simulink model "problem1_model"  (R2023b)
settings: Solver=ode8  StartTime=0.0  StopTime=30  FixedStep=1e-3  RelTol=1e-3
values from neighbouring files (symbols this model uses):
  h = A_3    (= 2)    [plotting_from_sim.m]    (also in problem1.m; problem1_1.m; proj_cnl_exer_21.m = x1-x2)
  ic = 0    [plotting_from_sim.m]    (also in problem1.m; problem1_1.m)
  k = 2    [plotting_from_sim.m]    (also in problem1.m; problem1_1.m)
  M_2 = 1    [plotting_from_sim.m]    (also in problem1.m; problem1_1.m)
  M_3 = B_3    (= 0.5)    [plotting_from_sim.m]    (also in problem1.m; problem1_1.m)
  S_1 = A_1    (= 0.5)    [plotting_from_sim.m]    (also in problem1.m; problem1_1.m)
  S_2 = A_2    (= 1)    [plotting_from_sim.m]    (also in problem1.m; problem1_1.m)
settings Model: Creator=afons  LastModifiedBy=afons

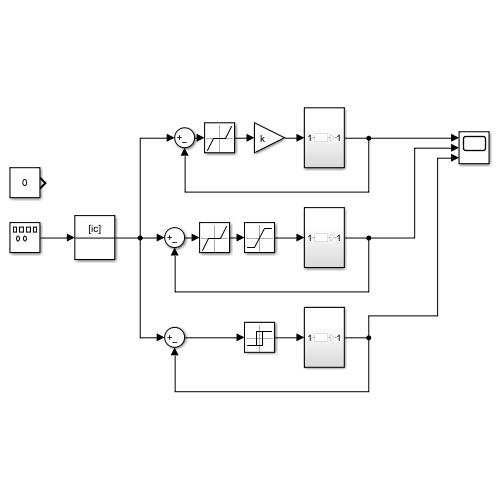
[thumbnail: Simulink's stored preview of the top-level diagram]
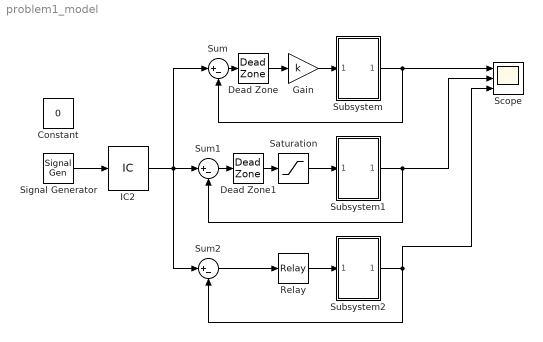
== system problem1_model ==
  Constant : Constant  Value=0
  Dead Zone : DeadZone  LowerValue=-S_1  UpperValue=S_1
  Dead Zone1 : DeadZone  LowerValue=-S_2  UpperValue=S_2
  Gain : Gain  Gain=k
  IC2 : InitialCondition  Value=ic
  Relay : Relay  OnSwitchValue=h  OffSwitchValue=-h  OnOutputValue=M_3  OffOutputValue=-M_3
  Saturation : Saturate  UpperLimit=M_2  LowerLimit=-M_2
  Scope : Scope  NumInputPorts=3
  Signal Generator : SignalGenerator  Frequency=0.5  Units=rad/sec
  Subsystem : Subsystem
  Subsystem1 : Subsystem
  Subsystem2 : Subsystem
  Sum : Sum  Inputs=|+-
  Sum1 : Sum  Inputs=|+-
  Sum2 : Sum  Inputs=|+-
  wires:
  Dead Zone1/1 -> Saturation/1
  Sum/1 -> Dead Zone/1
  Subsystem/1(Out1) -> Sum/2, Scope/1
  Subsystem1/1(Out1) -> Scope/2, Sum1/2
  Saturation/1 -> Subsystem1/1(In1)
  Sum1/1 -> Dead Zone1/1
  Subsystem2/1(Out1) -> Scope/3, Sum2/2
  Relay/1 -> Subsystem2/1(In1)
  Sum2/1 -> Relay/1
  Dead Zone/1 -> Gain/1
  Gain/1 -> Subsystem/1(In1)
  IC2/1 -> Sum/1, Sum2/1, Sum1/1
  Signal Generator/1 -> IC2/1

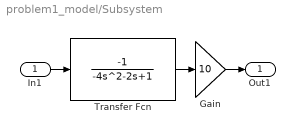
== system problem1_model/Subsystem ==
  In1 : Inport
  Gain : Gain  Gain=10
  Transfer Fcn : TransferFcn  Numerator=[-1]  Denominator=[-4 , -2 , 1]
  Out1 : Outport
  wires:
  Transfer Fcn/1 -> Gain/1
  In1/1 -> Transfer Fcn/1
  Gain/1 -> Out1/1

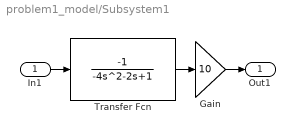
== system problem1_model/Subsystem1 ==
  In1 : Inport
  Gain : Gain  Gain=10
  Transfer Fcn : TransferFcn  Numerator=[-1]  Denominator=[-4 , -2 , 1]
  Out1 : Outport
  wires:
  Transfer Fcn/1 -> Gain/1
  In1/1 -> Transfer Fcn/1
  Gain/1 -> Out1/1

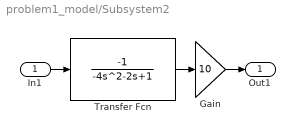
== system problem1_model/Subsystem2 ==
  In1 : Inport
  Gain : Gain  Gain=10
  Transfer Fcn : TransferFcn  Numerator=[-1]  Denominator=[-4 , -2 , 1]
  Out1 : Outport
  wires:
  Transfer Fcn/1 -> Gain/1
  In1/1 -> Transfer Fcn/1
  Gain/1 -> Out1/1
